simulink model "AFASClosedloopSim"  (R2023a)
settings: Solver=FixedStepAuto  StartTime=0.0  StopTime=600  FixedStep=1/240  RelTol=1e-5
PreLoadFcn:
  | [aircraft, state] = astDehavillandBeaver();
  | thrustX = getCoefficient(aircraft,"CX","Propeller",Component="Propeller");
InitFcn:
  | AFASClosedloopSimInitialization
model workspace (MATLAB code in the model file + MAT data in the model file):
  AirReferencedVelocity = 1
  AircraftPerformance : object (value not decoded)
  CurrentWaypoint = 1
  FCCLatDirMode = 1
  FCCVerticalMode = 1
  FlightPlan = 1
  LookaheadDis = 15
  NextWaypoint = 1
  NumofWaypoint = 1
  OwnshipAircraftID = 1
  PreWaypoint = 1
  PreviousWaypoint : Simulink.Parameter (value not decoded)
  TrajectoryChange = 1
  WaypointType = 1
  inputs0 : object (value not decoded)
  states : object (value not decoded)
  states0 : object (value not decoded)
  other statements: initialize6DOFSkyHogg;
values from neighbouring files (symbols this model uses):
  alt_ft = 1000    [AFASClosedloopSimInitialization.m]
  alt_hold_av = 1.5    [AFASClosedloopSimInitialization.m]
  alt_hold_hold = 0.1    [AFASClosedloopSimInitialization.m]
  alt_hold_vs = 0.58    [AFASClosedloopSimInitialization.m]
  alt_m = 304.8    [AFASClosedloopSimInitialization.m]
  AT_lead_T1 = 1    [AFASClosedloopSimInitialization.m]
  AT_lead_T2 = 1    [AFASClosedloopSimInitialization.m]
  AT_spd_hold_cmpst = 0.5    [AFASClosedloopSimInitialization.m]
  AT_spd_hold_ptch_tau_gain = 0.15    [AFASClosedloopSimInitialization.m]
  AT_spd_hold_rate_damping_gain = 10    [AFASClosedloopSimInitialization.m]
  AT_spd_hold_tas_lp_tau = 5.0    (= 5)    [AFASClosedloopSimInitialization.m]
  AT_spd_hold_tas_val_lp_tau = 0.5    [AFASClosedloopSimInitialization.m]
  AT_struct_den = 1    [AFASClosedloopSimInitialization.m]
  AT_struct_num = 1    [AFASClosedloopSimInitialization.m]
  AT_svo_composite = 1    [AFASClosedloopSimInitialization.m]
  av_hp_fltr_tau = 10    [AFASClosedloopSimInitialization.m]
  av_lp_fltr_tau = 0.5    [AFASClosedloopSimInitialization.m]
  cas_mps = 72.0222    [AFASClosedloopSimInitialization.m]
  Cl0 = 5.910000000000000e-04    (= 0.000591)    [AFASClosedloopSimInitialization.m]
  Cl_beta = -0.0618    [AFASClosedloopSimInitialization.m]
  Cl_da = -0.0992    [AFASClosedloopSimInitialization.m]
  Cl_da_alpha = -0.0827    [AFASClosedloopSimInitialization.m]
  Cl_dr = 0.0069    [AFASClosedloopSimInitialization.m]
  Cl_p = -0.5045    [AFASClosedloopSimInitialization.m]
  Cl_r = 0.1695    [AFASClosedloopSimInitialization.m]
  Cm0 = 0.0945    [AFASClosedloopSimInitialization.m]
  Cm_alpha = -0.6028    [AFASClosedloopSimInitialization.m]
  Cm_alpha2 = -2.1400    (= -2.14)    [AFASClosedloopSimInitialization.m]
  Cm_beta2 = 0.6921    [AFASClosedloopSimInitialization.m]
  Cm_de = -1.9210    (= -1.921)    [AFASClosedloopSimInitialization.m]
  Cm_df = 0.4072    [AFASClosedloopSimInitialization.m]
  Cm_q = -15.5600    (= -15.56)    [AFASClosedloopSimInitialization.m]
  Cm_r = -0.3118    [AFASClosedloopSimInitialization.m]
  Cn0 = -0.0031    [AFASClosedloopSimInitialization.m]
  Cn_beta = 0.0067    [AFASClosedloopSimInitialization.m]
  Cn_beta3 = 0.1373    [AFASClosedloopSimInitialization.m]
  Cn_da = -0.0039    [AFASClosedloopSimInitialization.m]
  Cn_dr = -0.0827    [AFASClosedloopSimInitialization.m]
  Cn_p = -0.1585    [AFASClosedloopSimInitialization.m]
  Cn_q = 0.1595    [AFASClosedloopSimInitialization.m]
  Cn_r = -0.1112    [AFASClosedloopSimInitialization.m]
  Cx0 = -0.0355    [AFASClosedloopSimInitialization.m]
  Cx_alpha = 0.0029    [AFASClosedloopSimInitialization.m]
  Cx_alpha2 = 5.4590    (= 5.459)    [AFASClosedloopSimInitialization.m]
  Cx_alpha3 = -5.1620    (= -5.162)    [AFASClosedloopSimInitialization.m]
  Cx_df = -0.0945    [AFASClosedloopSimInitialization.m]
  Cx_df_alpha = 1.1060    (= 1.106)    [AFASClosedloopSimInitialization.m]
  Cx_dr = 0.0341    [AFASClosedloopSimInitialization.m]
  Cx_q = -0.6748    [AFASClosedloopSimInitialization.m]
  Cy0 = -0.0022    [AFASClosedloopSimInitialization.m]
  Cy_beta = -0.7678    [AFASClosedloopSimInitialization.m]
  Cy_da = -0.0296    [AFASClosedloopSimInitialization.m]
  Cy_dr = 0.1158    [AFASClosedloopSimInitialization.m]
  Cy_dr_alpha = 0.5238    [AFASClosedloopSimInitialization.m]
  Cy_p = -0.1240    (= -0.124)    [AFASClosedloopSimInitialization.m]
  Cy_r = 0.3666    [AFASClosedloopSimInitialization.m]
  Cz0 = -0.0550    (= -0.055)    [AFASClosedloopSimInitialization.m]
  Cz_alpha = -5.5780    (= -5.578)    [AFASClosedloopSimInitialization.m]
  Cz_alpha3 = 3.4420    (= 3.442)    [AFASClosedloopSimInitialization.m]
  Cz_de = -0.3980    (= -0.398)    [AFASClosedloopSimInitialization.m]
  Cz_de_beta = -15.9300    (= -15.93)    [AFASClosedloopSimInitialization.m]
  Cz_df = -1.3770    (= -1.377)    [AFASClosedloopSimInitialization.m]
  Cz_df_alpha = -1.2610    (= -1.261)    [AFASClosedloopSimInitialization.m]
  Cz_q = -2.9880    (= -2.988)    [AFASClosedloopSimInitialization.m]
  hdg_select_hdg_rate_capt = 0.2    [AFASClosedloopSimInitialization.m]
  hdg_select_hdg_rate_damping = 1    [AFASClosedloopSimInitialization.m]
  hdg_select_hdg_rate_track = 0.05    [AFASClosedloopSimInitialization.m]
  lat_accel_aug_lp_tau = 10    [AFASClosedloopSimInitialization.m]
  ltrl_acc_gain = -0.04    [AFASClosedloopSimInitialization.m]
  ltrl_acc_lp_tau = 0.5    [AFASClosedloopSimInitialization.m]
  mach = 0.213    [AFASClosedloopSimInitialization.m]
  OwnshipAircraftConfig = 0    [AFASClosedloopSimInitialization.m]
  pitch_att_gain = 0.7    [AFASClosedloopSimInitialization.m]
  pitch_lead_T1 = 1    [AFASClosedloopSimInitialization.m]
  pitch_lead_T2 = 1    [AFASClosedloopSimInitialization.m]
  pitch_rate_gain = -1400    [AFASClosedloopSimInitialization.m]
  pitch_rate_gain_GAIN1 = -56    [AFASClosedloopSimInitialization.m]
  pitch_rate_gain_GAIN2 = -52.25    [AFASClosedloopSimInitialization.m]
  pitch_rate_gain_IAS1 = 100    [AFASClosedloopSimInitialization.m]
  pitch_rate_gain_IAS2 = 380    [AFASClosedloopSimInitialization.m]
  pitch_rate_gain_schd = [4.24        2.80        2.24        1.68        1.44        1.22        0.97        0.85        0.77        0.72        0.66    ] * 1000    [AFASClosedloopSimInitialization.m]
  pitch_rate_gain_spd = [85          100.0       120.00      140.00      160.00      180.00      200.00      220.00      240.00      260.00      275.00  ] * 0.5144444    [AFASClosedloopSimInitialization.m]
  pitch_schedule_type = 3    [AFASClosedloopSimInitialization.m]
  pitch_struct_den = 1    [AFASClosedloopSimInitialization.m]
  pitch_struct_num = 1    [AFASClosedloopSimInitialization.m]
  pitch_svo_composite = 1    [AFASClosedloopSimInitialization.m]
  pitch_svo_integral = 0.6    [AFASClosedloopSimInitialization.m]
  roll_att_gain = 0.45    [AFASClosedloopSimInitialization.m]
  roll_lead_T1 = 1    [AFASClosedloopSimInitialization.m]
  roll_lead_T2 = 1    [AFASClosedloopSimInitialization.m]
  roll_limit = 30*d2r    (= 0.5235987)    [AFASClosedloopSimInitialization.m]
  roll_rate_gain = 561.5    [AFASClosedloopSimInitialization.m]
  roll_rate_gain_GAIN1 = 57.25    [AFASClosedloopSimInitialization.m]
  roll_rate_gain_GAIN2 = 41.25    [AFASClosedloopSimInitialization.m]
  roll_rate_gain_IAS1 = 100    [AFASClosedloopSimInitialization.m]
  roll_rate_gain_IAS2 = 380    [AFASClosedloopSimInitialization.m]
  roll_rate_gain_schd = [1.30        0.86        0.71        0.63        0.57        0.50        0.46        0.46    ] * 1000    [AFASClosedloopSimInitialization.m]
  roll_rate_gain_spd = [85.00       100.00      120.00      140.00      160.00      200.00      220.00      275.00  ] * 0.5144444    [AFASClosedloopSimInitialization.m]
  roll_schedule_type = 3    [AFASClosedloopSimInitialization.m]
  roll_struct_den = 1    [AFASClosedloopSimInitialization.m]
  roll_struct_num = 1    [AFASClosedloopSimInitialization.m]
  roll_svo_composite = 0.00001    (= 1e-05)    [AFASClosedloopSimInitialization.m]
  roll_svo_integral = 0.6    [AFASClosedloopSimInitialization.m]
  tas_mps = 73.051    [AFASClosedloopSimInitialization.m]
  TGR = 0.25    [AFASClosedloopSimInitialization.m]
  wingrock_enable_alt = 20000    [AFASClosedloopSimInitialization.m]
  wingrock_enable_mach = 0.6    [AFASClosedloopSimInitialization.m]
  wingrock_lookup_data = [2 2  1 1]    [AFASClosedloopSimInitialization.m]
  wingrock_lookup_row = [0 2 5 10]*pi/180    [AFASClosedloopSimInitialization.m]
  wingrock_schedule_type = 3    [AFASClosedloopSimInitialization.m]
  yaw_rate_gain = 15521    [AFASClosedloopSimInitialization.m]
  yaw_rate_gain_GAIN1 = 37.8352    [AFASClosedloopSimInitialization.m]
  yaw_rate_gain_GAIN2 = 24.2654    [AFASClosedloopSimInitialization.m]
  yaw_rate_gain_IAS1 = 100    [AFASClosedloopSimInitialization.m]
  yaw_rate_gain_IAS2 = 340    [AFASClosedloopSimInitialization.m]
  yaw_rate_gain_piecewise_schd = [7.68	5.98		3.22	2.59		1.78 ... (first row only)    [AFASClosedloopSimInitialization.m]
  yaw_rate_gain_schd = [15521    11532   11532   10115   8951.7  7831.7  6829.2  5739.3  4506.7  3317.9  3391.5  2103.9  1404.5  994.3226]    [AFASClosedloopSimInitialization.m]
  yaw_rate_gain_spd = [90       97      106     111     118     127     136     149     165     187     192     228     264     295     ] * 0.5144444    [AFASClosedloopSimInitialization.m]
  yaw_rate_hp_tau = 1.8    [AFASClosedloopSimInitialization.m]
  yd_lead_T1 = yd_a * yd_lead_T2    [AFASClosedloopSimInitialization.m]
  ... (+7 more)
undefined symbols (not defined in the file or in its folder): aircraft, DiscIntNeverNeededParam, Earth, F, Light, MIL, sigbuilder_block, state, WGS84
libraries: aerolibasang x4, aerolibactuator x4, aerolibguid x2, simulink x2, dspnetwork x2, etargetslib x2, shared6dof x1, aerolibadyn x1, aerolibatmos2 x1, aerolibwind2 x1, aerolibtransform2 x1, sharedtransform x1
(part 4 of 4)

== system AFASClosedloopSim/FMGC (Flight Mgt and Guidance & Control)/AFCC: Albatross.ai Flight Control Computer/FCC: Outerloop & Innerloop Control Laws/HDG Mode/Outerloop Control Law ==
  psiCmd_rad : Inport
  psiF_rad : Inport  Port=2
  psiDotF_rps : Inport  Port=3
  "phiF_rad " : Inport  Port=4
  "phiDotF_rps " : Inport  Port=5
  rF_rps : Inport  Port=6
  "AyF_mpss " : Inport  Port=7
  Constant : Constant  Value=tas_mps
      settings: AttributesFormatString=TAS_mps
  HDG Flight Director : Subsystem
  Manual Switch4 : ManualSwitch  CurrentSetting=0
  Outerloop AP Delay{,1..3} (4 alike) : TransportDelay  DelayTime=0.004
  Outerloop FD Delay : TransportDelay  DelayTime=0.0905
  PFD/MFD Delay1 : TransportDelay  DelayTime=0.0175
  PFD/MFD Delay2 : TransportDelay  DelayTime=0.0175
  PFD/MFD Delay3 : TransportDelay  DelayTime=0.0175
  Roll Command Ay Augmentation : Subsystem
  Scope1 : Scope
  Scope2 : Scope
  Subsystem1 : Subsystem  mask(Zero-Order Hold){Tau=0.025}
      mask prompts: Tau "Tau (s)"
      mask help: Zero-Order Hold
      settings: AttributesFormatString=ZOH\n
      mask Display: disp([num2str(1/Tau),'Hz'])
  Subsystem2 : Subsystem  mask(Zero-Order Hold){Tau=0.025}
      mask prompts: Tau "Tau (s)"
      mask help: Zero-Order Hold
      settings: AttributesFormatString=ZOH\n
      mask Display: disp([num2str(1/Tau),'Hz'])
  Subsystem3 : Subsystem  mask(Zero-Order Hold){Tau=0.025}
      mask prompts: Tau "Tau (s)"
      mask help: Zero-Order Hold
      settings: AttributesFormatString=ZOH\n
      mask Display: disp([num2str(1/Tau),'Hz'])
  Subsystem4 : Subsystem  mask(Zero-Order Hold){Tau=0.025}
      mask prompts: Tau "Tau (s)"
      mask help: Zero-Order Hold
      settings: AttributesFormatString=ZOH\n
      mask Display: disp([num2str(1/Tau),'Hz'])
  Subsystem5 : Subsystem  mask(Zero-Order Hold){Tau=0.1000}
      mask prompts: Tau "Tau (s)"
      mask help: Zero-Order Hold
      settings: AttributesFormatString=ZOH\n
      mask Display: disp([num2str(1/Tau),'Hz'])
  Sum : Sum  Inputs=|++  SaturateOnIntegerOverflow=on
  hdg_select : Subsystem
  phiCmd_rad : Outport  InitialOutput=0
  phiC_rad : Outport  Port=2
  rC_rps : Outport  Port=3
  AyC_mpss : Outport  Port=4
  phiDotC_rps : Outport  Port=5
  wires:
  HDG Flight Director/1(phiCmd_rad) -> Manual Switch4/2
  "phiF_rad "/1 -> Outerloop AP Delay1/1
  "phiDotF_rps "/1 -> Outerloop AP Delay3/1
  rF_rps/1 -> Outerloop AP Delay2/1
  "AyF_mpss "/1 -> Outerloop AP Delay/1, PFD/MFD Delay3/1
  Subsystem5/1(Out) -> Scope2/1, phiCmd_rad/1
  Outerloop AP Delay2/1 -> Subsystem3/1(In)
  Subsystem4/1(Out) -> AyC_mpss/1
  Subsystem1/1(Out) -> phiC_rad/1
  Subsystem2/1(Out) -> phiDotC_rps/1
  Subsystem3/1(Out) -> rC_rps/1
  Outerloop AP Delay/1 -> Subsystem4/1(In)
  Outerloop AP Delay3/1 -> Subsystem2/1(In)
  Outerloop AP Delay1/1 -> Subsystem1/1(In)
  PFD/MFD Delay2/1 -> HDG Flight Director/2(psi_rad), hdg_select/2(hdg)
  PFD/MFD Delay3/1 -> Roll Command Ay Augmentation/1(AyAHF_m)
  Outerloop FD Delay/1 -> Subsystem5/1(In)
  psiDotF_rps/1 -> PFD/MFD Delay1/1
  PFD/MFD Delay1/1 -> HDG Flight Director/3(psiDot_rps), hdg_select/4(hdg_rate)
  Sum/1 -> Outerloop FD Delay/1
  Roll Command Ay Augmentation/1(augCmd_rad) -> Sum/2
  psiCmd_rad/1 -> Scope1/1, HDG Flight Director/1(psiCmd_rad), hdg_select/1(slctd_hdg)
  Constant/1 -> hdg_select/3(tas)
  hdg_select/1(roll_cmd) -> Manual Switch4/1
  Manual Switch4/1 -> Sum/1
  psiF_rad/1 -> PFD/MFD Delay2/1

== system AFASClosedloopSim/FMGC (Flight Mgt and Guidance & Control)/AFCC: Albatross.ai Flight Control Computer/FCC: Outerloop & Innerloop Control Laws/ALT Mode/Innerloop Control Law/Autopilot IAS-scheduled Gain ==
  ias : Inport
  Gain Sign : Constant  Value=-1
  Look-Up Table : Lookup  InputValues="[ias_1  ias_2]"  Table="[abs_gain_1  abs_gain_2]"  LookUpMeth=Interpolation-Use End Values
  Product : Product  InputSameDT=on  SaturateOnIntegerOverflow=on  OutDataTypeStr=Inherit: Same as first input
  dB->linear : Fcn  Expr=2^(u(1)/8)
  scheduled_gain : Outport
  wires:
  Gain Sign/1 -> Product/2
  Product/1 -> scheduled_gain/1
  ias/1 -> Look-Up Table/1
  dB->linear/1 -> Product/1
  Look-Up Table/1 -> dB->linear/1

== system AFASClosedloopSim/FMGC (Flight Mgt and Guidance & Control)/AFCC: Albatross.ai Flight Control Computer/FCC: Outerloop & Innerloop Control Laws/ALT Mode/Outerloop Control Law/Alt Upset_m ==
  Demux : Demux  Tag=STV Demux  Outputs=1
      settings: DisplayOption=none
  FromWs : FromWorkspace  Tag=STV FromWs  VariableName=tuvar
      SigBuilderData=|
      | common.afterFinalStr = 'Extrapolate'
      | common.sampleTime = 0
      | dataSet.timeRange = [0 50]
      | dataSet.name = 'Group 1'
      | sbobj.Groups.Name = 'Group 1'
      | sbobj.Groups.Signals.Name = 'Signal 2'
      | sbobj.Groups.Signals.XData = [0 5 5 6 6 50]
      | sbobj.Groups.Signals.YData = [0 0 5 5 0 0]
      | sbobj.Groups.TimeRange = [0 50]
  Signal 2 : Outport  Tag=STV Outport
  wires:
  Demux/1 -> Signal 2/1
  FromWs/1 -> Demux/1

== system AFASClosedloopSim/FMGC (Flight Mgt and Guidance & Control)/AFCC: Albatross.ai Flight Control Computer/FCC: Outerloop & Innerloop Control Laws/ALT Mode/Outerloop Control Law/Complementary Filter ==
  hd_mps : Inport
  hdd_mpss : Inport  Port=2
  " Av_HP" : TransferFcn  Numerator=[1 0]  Denominator=[av_hp_fltr_tau 1]
  " HP Filter  " : TransferFcn  Numerator=[1.2596 2.0202]  Denominator=[1.2596 2.0202 1]
  HP Filter : TransferFcn  Numerator=[1.2596 2.0202]  Denominator=[1.2596 2.0202 1]
  Sum1 : Sum  Inputs=++|  SaturateOnIntegerOverflow=on
  Sum2 : Sum  Inputs=|++  SaturateOnIntegerOverflow=on
  Sum3 : Sum  Inputs=++|  SaturateOnIntegerOverflow=on
  av_hp_fltr_tau : Gain  Gain=av_hp_fltr_tau  SaturateOnIntegerOverflow=on  OutDataTypeStr=Inherit: Same as input  ParamDataTypeStr=Inherit: Same as input
  hdF_mps : Outport
  hddF_mpss : Outport  Port=2
  wires:
  hdd_mpss/1 -> HP Filter/1, av_hp_fltr_tau/1
  hd_mps/1 -> Sum1/1, Sum3/1
  Sum2/1 -> Sum3/2
  HP Filter/1 -> Sum2/1
  av_hp_fltr_tau/1 -> Sum2/2
  Sum1/1 -> hdF_mps/1
  " HP Filter  "/1 -> Sum1/2
  " Av_HP"/1 -> " HP Filter  "/1, hddF_mpss/1
  Sum3/1 -> " Av_HP"/1

== system AFASClosedloopSim/FMGC (Flight Mgt and Guidance & Control)/AFCC: Albatross.ai Flight Control Computer/FCC: Outerloop & Innerloop Control Laws/ALT Mode/Outerloop Control Law/Subsystem ==
  In : Inport
  ZOH : TransferFcn  Numerator=[-Tau/6 1]  Denominator=[Tau/3 1]
  Out : Outport
  wires:
  ZOH/1 -> Out/1
  In/1 -> ZOH/1

== system AFASClosedloopSim/FMGC (Flight Mgt and Guidance & Control)/AFCC: Albatross.ai Flight Control Computer/FCC: Outerloop & Innerloop Control Laws/ALT Mode/Outerloop Control Law/Subsystem1 ==
  In : Inport
  ZOH : TransferFcn  Numerator=[-Tau/6 1]  Denominator=[Tau/3 1]
  Out : Outport
  wires:
  In/1 -> ZOH/1
  ZOH/1 -> Out/1

== system AFASClosedloopSim/FMGC (Flight Mgt and Guidance & Control)/AFCC: Albatross.ai Flight Control Computer/FCC: Outerloop & Innerloop Control Laws/ALT Mode/Outerloop Control Law/VS Upset_fpm ==
  Demux : Demux  Tag=STV Demux  Outputs=1
      settings: DisplayOption=none
  FromWs : FromWorkspace  Tag=STV FromWs  VariableName=tuvar
      SigBuilderData=|
      | common.afterFinalStr = 'Extrapolate'
      | common.sampleTime = 0
      | dataSet.timeRange = [0 50]
      | dataSet.name = 'Group 1'
      | sbobj.Groups.Name = 'Group 1'
      | sbobj.Groups.Signals.Name = 'Signal 2'
      | sbobj.Groups.Signals.XData = [0 5 5 6 6 50]
      | sbobj.Groups.Signals.YData = [0 0 200 200 0 0]
      | sbobj.Groups.TimeRange = [0 50]
  Signal 2 : Outport  Tag=STV Outport
  wires:
  FromWs/1 -> Demux/1
  Demux/1 -> Signal 2/1

== system AFASClosedloopSim/FMGC (Flight Mgt and Guidance & Control)/AFCC: Albatross.ai Flight Control Computer/FCC: Outerloop & Innerloop Control Laws/Autothrottle/AT SPD Hold//Select/Subsystem ==
  In : Inport
  ZOH : TransferFcn  Numerator=[-Tau/6 1]  Denominator=[Tau/3 1]
  Out : Outport
  wires:
  ZOH/1 -> Out/1
  In/1 -> ZOH/1

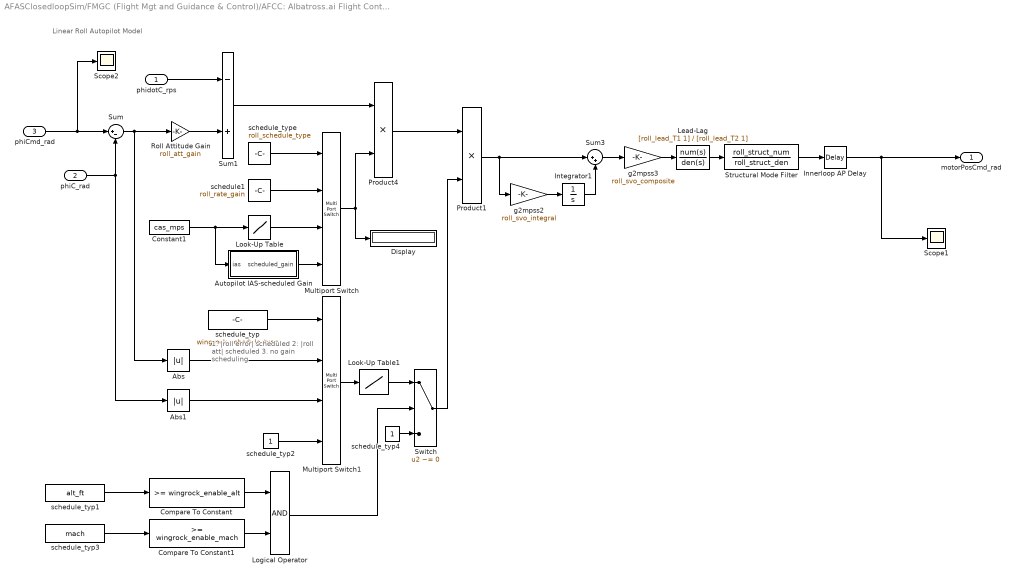
== system AFASClosedloopSim/FMGC (Flight Mgt and Guidance & Control)/AFCC: Albatross.ai Flight Control Computer/FCC: Outerloop & Innerloop Control Laws/HDG Mode/Innerloop Control Law/Roll AP ==
  note: Linear Roll Autopilot Model
  note: 1: |roll error| scheduled
      | 2: |roll att| scheduled
      | 3. no gain scheduling
  phidotC_rps : Inport
  phiC_rad : Inport  Port=2
  phiCmd_rad : Inport  Port=3
  Abs : Abs  SaturateOnIntegerOverflow=off
  Abs1 : Abs  SaturateOnIntegerOverflow=off
  Autopilot IAS-scheduled Gain : Subsystem  mask(Autopilot IAS-scheduled Gain){IAS1=roll_rate_gain_IAS1, IAS2=roll_rate_gain_IAS2, GAIN1=roll_rate_gain_GAIN1, GAIN2=roll_rate_gain_GAIN2}
      mask prompts: IAS1 "IAS1 (lower IAS limit, knots)"; IAS2 "IAS2 (upper IAS limit, knots)"; GAIN1 "GAIN1 (the gain for IAS1, dB)"; GAIN2 "GAIN2 (the gain for IAS2, dB)"
      mask help:
      | Autopilot gain scheduling based on the indicated airspeed.
      |
      | Parameters:
      | IAS1 (lower IAS limit, knots)  -- lower IAS limit (unit: knot)
      | IAS2 (upper IAS limit, knots) -- upper IAS limit (unit: knot)
      | GAIN1 (the gain for IAS1, dB) -- the gain for the lower IAS limit (unit: dB)
      | GAIN2 (the gain for IAS2, dB) -- the gain for the upper IAS limit (unit: dB)
      |
      | Inputs:
      | ias -- indicated airspeed (unit: meter/second)
      |
      | Outputs:
      | scheduled_gain -- indicated airspeed scheduled gain
      mask init:
      | ias_1 = IAS1 * 0.5144444;
      | ias_2 = IAS2 * 0.5144444;
      | abs_gain_1 = abs( GAIN1 ) * 8 / 6;
      | abs_gain_2 = abs( GAIN2 ) * 8 / 6;
      | gain_sign = sign( GAIN1 );
      mask Help:
      | Autopilot gain scheduling based on the indicated airspeed.
      | 
      | Parameters:
      | IAS1 (lower IAS limit, knots)  -- lower IAS limit (unit: knot)
      | IAS2 (upper IAS limit, knots) -- upper IAS limit (unit: knot)
      | GAIN1 (the gain for IAS1, dB) -- the gain for the lower IAS limit (unit: dB)
      | GAIN2 (the gain for IAS2, dB) -- the gain for the upper IAS limit (unit: dB)
      | 
      | Inputs:
      | ias -- indicated airspeed (unit: meter/second)
      | 
      | Outputs:
      | scheduled_gain -- indicated airspeed scheduled gain
  Compare To Constant : simulink/Logic and Bit Operations/Compare To Constant  relop=>=  const=wingrock_enable_alt  OutDataTypeStr=boolean
  Compare To Constant1 : simulink/Logic and Bit Operations/Compare To Constant  relop=>=  const=wingrock_enable_mach  OutDataTypeStr=boolean
  Constant1 : Constant  Value=cas_mps
      settings: AttributesFormatString=CAS_mps
  Display : Display
  Innerloop AP Delay : TransportDelay  DelayTime=0.003
  Integrator1 : Integrator
  Lead-Lag : TransferFcn  Numerator=[roll_lead_T1 1]  Denominator=[roll_lead_T2 1]
  Logical Operator : Logic  AllPortsSameDT=off  OutDataTypeStr=boolean
  Look-Up Table : Lookup  InputValues=roll_rate_gain_spd  Table=roll_rate_gain_schd  LookUpMeth=Interpolation-Use End Values
  Look-Up Table1 : Lookup  InputValues=wingrock_lookup_row  Table=wingrock_lookup_data  LookUpMeth=Interpolation-Use End Values
  Multiport Switch : MultiPortSwitch  InputSameDT=off
  Multiport Switch1 : MultiPortSwitch  InputSameDT=off
  Product1 : Product  Inputs=**  InputSameDT=on  SaturateOnIntegerOverflow=on  OutDataTypeStr=Inherit: Same as first input
  Product4 : Product  Inputs=**  InputSameDT=on  SaturateOnIntegerOverflow=on  OutDataTypeStr=Inherit: Same as first input
  Roll Attitude Gain : Gain  Gain=roll_att_gain  SaturateOnIntegerOverflow=on  OutDataTypeStr=Inherit: Same as input  ParamDataTypeStr=Inherit: Same as input
      settings: AttributesFormatString=%<Gain>
  Scope1 : Scope
  Scope2 : Scope
  Structural Mode Filter : TransferFcn  Numerator=roll_struct_num  Denominator=roll_struct_den
  Sum : Sum  Inputs=|+-  SaturateOnIntegerOverflow=on
  Sum1 : Sum  Inputs=-+  SaturateOnIntegerOverflow=on
  Sum3 : Sum  Inputs=|++  SaturateOnIntegerOverflow=on
  Switch : Switch  Criteria=u2 ~= 0  SaturateOnIntegerOverflow=off  InputSameDT=off
  g2mpss2 : Gain  Gain=roll_svo_integral  SaturateOnIntegerOverflow=on  OutDataTypeStr=Inherit: Same as input  ParamDataTypeStr=Inherit: Same as input
  g2mpss3 : Gain  Gain=roll_svo_composite  SaturateOnIntegerOverflow=on  OutDataTypeStr=Inherit: Same as input  ParamDataTypeStr=Inherit: Same as input
  schedule1 : Constant  Value=roll_rate_gain
      settings: AttributesFormatString=roll_rate_gain
  schedule_typ : Constant  Value=wingrock_schedule_type
  schedule_typ1 : Constant  Value=alt_ft
  schedule_typ2 : Constant
  schedule_typ3 : Constant  Value=mach
  schedule_typ4 : Constant
  schedule_type : Constant  Value=roll_schedule_type
  motorPosCmd_rad : Outport
  wires:
  Sum1/1 -> Product4/1
  Roll Attitude Gain/1 -> Sum1/2
  Innerloop AP Delay/1 -> Scope1/1, motorPosCmd_rad/1
  Structural Mode Filter/1 -> Innerloop AP Delay/1
  Multiport Switch/1 -> Product4/2, Display/1
  Constant1/1 -> Autopilot IAS-scheduled Gain/1(ias), Look-Up Table/1
  schedule1/1 -> Multiport Switch/2
  Look-Up Table/1 -> Multiport Switch/3
  schedule_type/1 -> Multiport Switch/1
  Autopilot IAS-scheduled Gain/1(scheduled_gain) -> Multiport Switch/4
  Sum/1 -> Roll Attitude Gain/1, Abs/1
  Integrator1/1 -> Sum3/2
  g2mpss2/1 -> Integrator1/1
  Sum3/1 -> g2mpss3/1
  phiCmd_rad/1 -> Scope2/1, Sum/1
  phiC_rad/1 -> Sum/2, Abs1/1
  schedule_typ/1 -> Multiport Switch1/1
  schedule_typ2/1 -> Multiport Switch1/4
  schedule_typ1/1 -> Compare To Constant/1
  schedule_typ3/1 -> Compare To Constant1/1
  Compare To Constant/1 -> Logical Operator/1
  Compare To Constant1/1 -> Logical Operator/2
  Multiport Switch1/1 -> Look-Up Table1/1
  Logical Operator/1 -> Switch/2
  Look-Up Table1/1 -> Switch/1
  schedule_typ4/1 -> Switch/3
  Switch/1 -> Product1/2
  Product4/1 -> Product1/1
  Product1/1 -> Sum3/1, g2mpss2/1
  g2mpss3/1 -> Lead-Lag/1
  Lead-Lag/1 -> Structural Mode Filter/1
  phidotC_rps/1 -> Sum1/1
  Abs/1 -> Multiport Switch1/2
  Abs1/1 -> Multiport Switch1/3

== system AFASClosedloopSim/FMGC (Flight Mgt and Guidance & Control)/AFCC: Albatross.ai Flight Control Computer/FCC: Outerloop & Innerloop Control Laws/HDG Mode/Innerloop Control Law/YD Control Law ==
  phiC_rad : Inport
  rC_rps : Inport  Port=2
  AyC_mpss : Inport  Port=3
  Attitude Gain1 : Gain  Gain=ltrl_acc_gain  SaturateOnIntegerOverflow=on  OutDataTypeStr=Inherit: Same as input  ParamDataTypeStr=Inherit: Same as input
      settings: AttributesFormatString=%<Gain>
  Autopilot IAS-scheduled Gain : Subsystem  mask(Autopilot IAS-scheduled Gain){IAS1=yaw_rate_gain_IAS1, IAS2=yaw_rate_gain_IAS2, GAIN1=yaw_rate_gain_GAIN1, GAIN2=yaw_rate_gain_GAIN2}
      mask prompts: IAS1 "IAS1 (lower IAS limit, knots)"; IAS2 "IAS2 (upper IAS limit, knots)"; GAIN1 "GAIN1 (the gain for IAS1, dB)"; GAIN2 "GAIN2 (the gain for IAS2, dB)"
      mask help:
      | Autopilot gain scheduling based on the indicated airspeed.
      |
      | Parameters:
      | IAS1 (lower IAS limit, knots)  -- lower IAS limit (unit: knot)
      | IAS2 (upper IAS limit, knots) -- upper IAS limit (unit: knot)
      | GAIN1 (the gain for IAS1, dB) -- the gain for the lower IAS limit (unit: dB)
      | GAIN2 (the gain for IAS2, dB) -- the gain for the upper IAS limit (unit: dB)
      |
      | Inputs:
      | ias -- indicated airspeed (unit: meter/second)
      |
      | Outputs:
      | scheduled_gain -- indicated airspeed scheduled gain
      mask init:
      | ias_1 = IAS1 * 0.5144444;
      | ias_2 = IAS2 * 0.5144444;
      | abs_gain_1 = abs( GAIN1 ) * 8 / 6;
      | abs_gain_2 = abs( GAIN2 ) * 8 / 6;
      | gain_sign = sign( GAIN1 );
      mask Help:
      | Autopilot gain scheduling based on the indicated airspeed.
      | 
      | Parameters:
      | IAS1 (lower IAS limit, knots)  -- lower IAS limit (unit: knot)
      | IAS2 (upper IAS limit, knots) -- upper IAS limit (unit: knot)
      | GAIN1 (the gain for IAS1, dB) -- the gain for the lower IAS limit (unit: dB)
      | GAIN2 (the gain for IAS2, dB) -- the gain for the upper IAS limit (unit: dB)
      | 
      | Inputs:
      | ias -- indicated airspeed (unit: meter/second)
      | 
      | Outputs:
      | scheduled_gain -- indicated airspeed scheduled gain
  CAS_mps : Constant  Value=cas_mps
  CAS_mps1 : Constant  Value=cas_mps
  Display : Display
  Innerloop AP Delay : TransportDelay  DelayTime=0.003
  Integrator1 : Integrator
  Lead-Lag : TransferFcn  Numerator=[yd_lead_T1 1]  Denominator=[yd_lead_T2 1]
  Look-Up Table : Lookup  InputValues=yaw_rate_gain_spd  Table=yaw_rate_gain_schd  LookUpMeth=Interpolation-Use End Values
  Lookup Table (2-D) : Lookup2D  RowIndex=yaw_rate_gain_piecewise_alt  ColumnIndex=yaw_rate_gain_piecewise_spd  Table=yaw_rate_gain_piecewise_schd  LookUpMeth=Interpolation-Use End Values  SaturateOnIntegerOverflow=off  InputSameDT=off
  Multiport Switch : MultiPortSwitch  Inputs=4  InputSameDT=off
  Product : Product  Inputs=*/  InputSameDT=on  SaturateOnIntegerOverflow=on  OutDataTypeStr=Inherit: Same as first input
  Product3 : Product  Inputs=**  InputSameDT=on  SaturateOnIntegerOverflow=on  OutDataTypeStr=Inherit: Same as first input
  Structural Mode Filter : TransferFcn  Numerator=yd_struct_num  Denominator=yd_struct_den
  Sum1 : Sum  Inputs=--  SaturateOnIntegerOverflow=on
  Sum2 : Sum  Inputs=+-  SaturateOnIntegerOverflow=on
  Sum3 : Sum  Inputs=|++  SaturateOnIntegerOverflow=on
  Transfer Fcn1 : TransferFcn  Numerator=1  Denominator=[ltrl_acc_lp_tau 1]
      settings: AttributesFormatString=1/(tau*s+1)
  Transfer Fcn2 : TransferFcn  Numerator="[yaw_rate_hp_tau   0]"  Denominator="[yaw_rate_hp_tau   1]"
      settings: AttributesFormatString=(tau*s) / (tau*s+1)
  alt_m : Constant  Value=alt_m
  g2mpss : Gain  Gain=9.80665  SaturateOnIntegerOverflow=on  OutDataTypeStr=Inherit: Same as input  ParamDataTypeStr=Inherit: Same as input
      settings: AttributesFormatString=g2mpss
  g2mpss1 : Gain  Gain=yd_svo_integral  SaturateOnIntegerOverflow=on  OutDataTypeStr=Inherit: Same as input  ParamDataTypeStr=Inherit: Same as input
  g2mpss2 : Gain  Gain=yd_svo_composite  SaturateOnIntegerOverflow=on  OutDataTypeStr=Inherit: Same as input  ParamDataTypeStr=Inherit: Same as input
  schedule1 : Constant  Value=yaw_rate_gain
      settings: AttributesFormatString=yaw_rate_gain
  schedule_type : Constant  Value=yd_schedule_type
  motorPosCmd_rad : Outport  InitialOutput=0
  wires:
  phiC_rad/1 -> Product/1
  Product/1 -> g2mpss/1
  AyC_mpss/1 -> Attitude Gain1/1
  Innerloop AP Delay/1 -> motorPosCmd_rad/1
  Sum2/1 -> Transfer Fcn2/1
  schedule1/1 -> Multiport Switch/2
  Sum1/1 -> Product3/1
  Look-Up Table/1 -> Multiport Switch/3
  Multiport Switch/1 -> Display/1, Product3/2
  Autopilot IAS-scheduled Gain/1(scheduled_gain) -> Multiport Switch/4
  schedule_type/1 -> Multiport Switch/1
  Structural Mode Filter/1 -> Innerloop AP Delay/1
  Product3/1 -> g2mpss1/1, Sum3/1
  CAS_mps1/1 -> Lookup Table (2-D)/2, Autopilot IAS-scheduled Gain/1(ias), Look-Up Table/1
  Integrator1/1 -> Sum3/2
  g2mpss1/1 -> Integrator1/1
  Sum3/1 -> g2mpss2/1
  g2mpss2/1 -> Lead-Lag/1
  CAS_mps/1 -> Product/2
  Lookup Table (2-D)/1 -> Multiport Switch/5
  alt_m/1 -> Lookup Table (2-D)/1
  Lead-Lag/1 -> Structural Mode Filter/1
  Attitude Gain1/1 -> Transfer Fcn1/1
  rC_rps/1 -> Sum2/2
  Transfer Fcn2/1 -> Sum1/1
  Transfer Fcn1/1 -> Sum1/2
  g2mpss/1 -> Sum2/1

== system AFASClosedloopSim/FMGC (Flight Mgt and Guidance & Control)/AFCC: Albatross.ai Flight Control Computer/FCC: Outerloop & Innerloop Control Laws/HDG Mode/Outerloop Control Law/HDG Flight Director ==
  psiCmd_rad : Inport
  psi_rad : Inport  Port=2
  psiDot_rps : Inport  Port=3
  Attitude Gain1 : Gain  Gain=hdg_select_hdg_rate_track  SaturateOnIntegerOverflow=on  OutDataTypeStr=Inherit: Same as input  ParamDataTypeStr=Inherit: Same as input
      settings: AttributesFormatString=%<Gain>
  Attitude Gain2 : Gain  Gain=hdg_select_hdg_rate_damping  SaturateOnIntegerOverflow=on  OutDataTypeStr=Inherit: Same as input  ParamDataTypeStr=Inherit: Same as input
      settings: AttributesFormatString=%<Gain>
  Attitude Gain3 : Gain  Gain=0.1020  SaturateOnIntegerOverflow=on  OutDataTypeStr=Inherit: Same as input  ParamDataTypeStr=Inherit: Same as input
      settings: AttributesFormatString=1/g
  Constant : Constant  Value=tas_mps
      settings: AttributesFormatString=TAS_mps
  Product : Product  SaturateOnIntegerOverflow=on  OutDataTypeStr=Inherit: Same as first input
  Sum1 : Sum  Inputs=|+-  SaturateOnIntegerOverflow=on
  Sum2 : Sum  Inputs=|+-  SaturateOnIntegerOverflow=on
  phiCmd_rad : Outport
  wires:
  Constant/1 -> Attitude Gain3/1
  Attitude Gain3/1 -> Product/2
  Attitude Gain1/1 -> Product/1
  psi_rad/1 -> Sum2/2
  Product/1 -> Sum1/1
  psiDot_rps/1 -> Attitude Gain2/1
  Attitude Gain2/1 -> Sum1/2
  Sum1/1 -> phiCmd_rad/1
  Sum2/1 -> Attitude Gain1/1
  psiCmd_rad/1 -> Sum2/1

== system AFASClosedloopSim/FMGC (Flight Mgt and Guidance & Control)/AFCC: Albatross.ai Flight Control Computer/FCC: Outerloop & Innerloop Control Laws/HDG Mode/Outerloop Control Law/Roll Command Ay Augmentation ==
  AyAHF_m : Inport
  Attitude Gain3 : Gain  Gain=0.1020  SaturateOnIntegerOverflow=on  OutDataTypeStr=Inherit: Same as input  ParamDataTypeStr=Inherit: Same as input
      settings: AttributesFormatString=1/g
  Gain1 : Gain  Gain=-1  SaturateOnIntegerOverflow=on  OutDataTypeStr=Inherit: Same as input  ParamDataTypeStr=Inherit: Same as input
      settings: AttributesFormatString=Flip Sign
  Transfer Fcn : TransferFcn  Denominator=[lat_accel_aug_lp_tau 1]
      settings: AttributesFormatString=Ay_LP
  augCmd_rad : Outport  InitialOutput=0
  wires:
  AyAHF_m/1 -> Gain1/1
  Attitude Gain3/1 -> Transfer Fcn/1
  Transfer Fcn/1 -> augCmd_rad/1
  Gain1/1 -> Attitude Gain3/1

== system AFASClosedloopSim/FMGC (Flight Mgt and Guidance & Control)/AFCC: Albatross.ai Flight Control Computer/FCC: Outerloop & Innerloop Control Laws/HDG Mode/Outerloop Control Law/Subsystem1 ==
  In : Inport
  ZOH : TransferFcn  Numerator=[-Tau/6 1]  Denominator=[Tau/3 1]
  Out : Outport
  wires:
  In/1 -> ZOH/1
  ZOH/1 -> Out/1

== system AFASClosedloopSim/FMGC (Flight Mgt and Guidance & Control)/AFCC: Albatross.ai Flight Control Computer/FCC: Outerloop & Innerloop Control Laws/HDG Mode/Outerloop Control Law/Subsystem2 ==
  In : Inport
  ZOH : TransferFcn  Numerator=[-Tau/6 1]  Denominator=[Tau/3 1]
  Out : Outport
  wires:
  ZOH/1 -> Out/1
  In/1 -> ZOH/1

== system AFASClosedloopSim/FMGC (Flight Mgt and Guidance & Control)/AFCC: Albatross.ai Flight Control Computer/FCC: Outerloop & Innerloop Control Laws/HDG Mode/Outerloop Control Law/Subsystem3 ==
  In : Inport
  ZOH : TransferFcn  Numerator=[-Tau/6 1]  Denominator=[Tau/3 1]
  Out : Outport
  wires:
  In/1 -> ZOH/1
  ZOH/1 -> Out/1

== system AFASClosedloopSim/FMGC (Flight Mgt and Guidance & Control)/AFCC: Albatross.ai Flight Control Computer/FCC: Outerloop & Innerloop Control Laws/HDG Mode/Outerloop Control Law/Subsystem4 ==
  In : Inport
  ZOH : TransferFcn  Numerator=[-Tau/6 1]  Denominator=[Tau/3 1]
  Out : Outport
  wires:
  ZOH/1 -> Out/1
  In/1 -> ZOH/1

== system AFASClosedloopSim/FMGC (Flight Mgt and Guidance & Control)/AFCC: Albatross.ai Flight Control Computer/FCC: Outerloop & Innerloop Control Laws/HDG Mode/Outerloop Control Law/Subsystem5 ==
  In : Inport
  ZOH : TransferFcn  Numerator=[-Tau/6 1]  Denominator=[Tau/3 1]
  Out : Outport
  wires:
  ZOH/1 -> Out/1
  In/1 -> ZOH/1

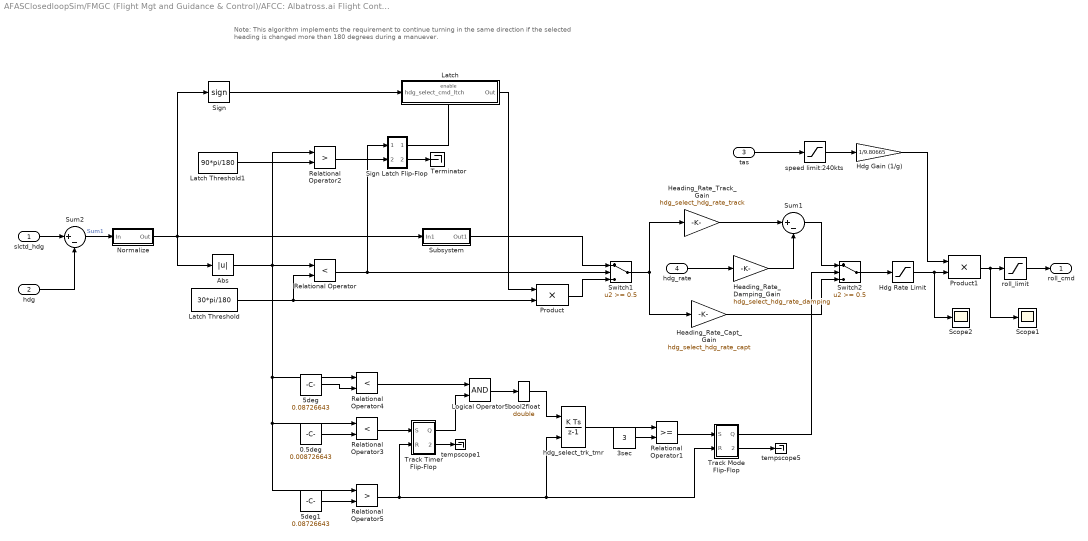
== system AFASClosedloopSim/FMGC (Flight Mgt and Guidance & Control)/AFCC: Albatross.ai Flight Control Computer/FCC: Outerloop & Innerloop Control Laws/HDG Mode/Outerloop Control Law/hdg_select ==
  note: Note: This algorithm implements the requirement to continue turning in the same direction
      |  if the selected heading is changed more than 180 degrees during a manuever.
  slctd_hdg : Inport
  hdg : Inport  Port=2
  tas : Inport  Port=3
  hdg_rate : Inport  Port=4
  0.5deg : Constant  Value=0.008726643
  3sec : Constant  Value=3
  5deg : Constant  Value=0.08726643
  5deg1 : Constant  Value=0.08726643
  Abs : Abs
  Hdg Gain (1/g) : Gain  Gain=1/9.80665  SaturateOnIntegerOverflow=on  OutDataTypeStr=Inherit: Same as input  ParamDataTypeStr=Inherit: Same as input
  Hdg Rate Limit : Saturate  UpperLimit=3*pi/180  LowerLimit=-3*pi/180
  Heading_Rate_Capt_Gain : Gain  Gain=hdg_select_hdg_rate_capt  SaturateOnIntegerOverflow=on  OutDataTypeStr=Inherit: Same as input  ParamDataTypeStr=Inherit: Same as input
  Heading_Rate_Damping_Gain : Gain  Gain=hdg_select_hdg_rate_damping  SaturateOnIntegerOverflow=on  OutDataTypeStr=Inherit: Same as input  ParamDataTypeStr=Inherit: Same as input
  Heading_Rate_Track_Gain : Gain  Gain=hdg_select_hdg_rate_track  SaturateOnIntegerOverflow=on  OutDataTypeStr=Inherit: Same as input  ParamDataTypeStr=Inherit: Same as input
  Latch : Subsystem  TreatAsAtomicUnit=on  RTWFcnName=HDGlatch  RTWFileName=testlatch
      settings: RTWSystemCode=Inline  RTWFcnNameOpts=User specified  RTWFileNameOpts=User specified
  Latch Threshold : Constant  Value=30*pi/180
  Latch Threshold1 : Constant  Value=90*pi/180
  Logical Operator5 : Logic  AllPortsSameDT=off
  Normalize : Subsystem  RTWFcnName=normalize
      settings: RTWFcnNameOpts=User specified
  Product : Product  SaturateOnIntegerOverflow=on  OutDataTypeStr=Inherit: Same as first input
  Product1 : Product  InputSameDT=on  SaturateOnIntegerOverflow=on  OutDataTypeStr=Inherit: Same as first input
  Relational Operator : RelationalOperator  Operator=<  InputSameDT=off
  Relational Operator1 : RelationalOperator  InputSameDT=off
  Relational Operator2 : RelationalOperator  Operator=>  InputSameDT=off
  Relational Operator3 : RelationalOperator  Operator=<  InputSameDT=off
  Relational Operator4 : RelationalOperator  Operator=<  InputSameDT=off
  Relational Operator5 : RelationalOperator  Operator=>  InputSameDT=off
  Scope1 : Scope
  Scope2 : Scope
  Sign : Signum
  Sign Latch Flip-Flop : Subsystem  AncestorBlock=simulink_extras/Flip Flops/S-R Flip-Flop  mask(SRFlipFlop){initial_condition=0}
      mask prompts: initial_condition "Initial condition (state of Q):"
      mask help: S-R Flip-Flop Block
      settings: LibrarySourceBlock=|
      | simulink_extras/Flip Flops/S-R
      | Flip-Flop
      mask Help:
      | The S-R flip-flop also known as a set-reset flip-flop. This implementation
      | is modeled after an S-R flip-flop constructed using NOR gates. The
      | truth table for this block is:
      | <pre>
      |  S  R   Q  !Q
      |  ----------------
      |  1  0   1  0
      |  0  0   1  0  (after S == 1, R == 0)
      |  0  1   0  1
      |  0  0   0  1  (after S == 0, R == 1)
      |  1  1   0  0
      | </pre>
      | 
      | In an S-R flip-flop that is implemented with NOR gates, when a 1 is
      | applied to both the set and reset inputs, both outputs go to 0. Technically,
      | this state is undefined and is usually avoided. Note, if the flip-flop is
      | implemented with NAND gates, when a 0 is applied to both inputs, both outputs
      | go to 0 and when a 1 is applied to both inputs, the output depends on
      | the previous state of the flip-flop (previous value of Q).
  Subsystem : Subsystem
  Sum1 : Sum  Inputs=|+-  InputSameDT=on  SaturateOnIntegerOverflow=on  OutDataTypeStr=Inherit: Same as first input
  Sum2 : Sum  Inputs=|+-  InputSameDT=on  SaturateOnIntegerOverflow=on  OutDataTypeStr=Inherit: Same as first input
  Switch1 : Switch  Threshold=0.5  InputSameDT=off
  Switch2 : Switch  Threshold=0.5  InputSameDT=off
  Terminator : Terminator
  Track Mode Flip-Flop : Subsystem  AncestorBlock=simulink_extras/Flip Flops/S-R Flip-Flop  mask(SRFlipFlop){initial_condition=0}
      mask prompts: initial_condition "Initial condition (state of Q):"
      mask help: S-R Flip-Flop Block
      settings: LibrarySourceBlock=|
      | simulink_extras/Flip Flops/S-R
      | Flip-Flop
      mask Help:
      | The S-R flip-flop also known as a set-reset flip-flop. This implementation
      | is modeled after an S-R flip-flop constructed using NOR gates. The
      | truth table for this block is:
      | <pre>
      |  S  R   Q  !Q
      |  ----------------
      |  1  0   1  0
      |  0  0   1  0  (after S == 1, R == 0)
      |  0  1   0  1
      |  0  0   0  1  (after S == 0, R == 1)
      |  1  1   0  0
      | </pre>
      | 
      | In an S-R flip-flop that is implemented with NOR gates, when a 1 is
      | applied to both the set and reset inputs, both outputs go to 0. Technically,
      | this state is undefined and is usually avoided. Note, if the flip-flop is
      | implemented with NAND gates, when a 0 is applied to both inputs, both outputs
      | go to 0 and when a 1 is applied to both inputs, the output depends on
      | the previous state of the flip-flop (previous value of Q).
  Track Timer Flip-Flop : Subsystem  AncestorBlock=simulink_extras/Flip Flops/S-R Flip-Flop  mask(SRFlipFlop){initial_condition=0}
      mask prompts: initial_condition "Initial condition (state of Q):"
      mask help: S-R Flip-Flop Block
      settings: LibrarySourceBlock=|
      | simulink_extras/Flip Flops/S-R
      | Flip-Flop
      mask Help:
      | The S-R flip-flop also known as a set-reset flip-flop. This implementation
      | is modeled after an S-R flip-flop constructed using NOR gates. The
      | truth table for this block is:
      | <pre>
      |  S  R   Q  !Q
      |  ----------------
      |  1  0   1  0
      |  0  0   1  0  (after S == 1, R == 0)
      |  0  1   0  1
      |  0  0   0  1  (after S == 0, R == 1)
      |  1  1   0  0
      | </pre>
      | 
      | In an S-R flip-flop that is implemented with NOR gates, when a 1 is
      | applied to both the set and reset inputs, both outputs go to 0. Technically,
      | this state is undefined and is usually avoided. Note, if the flip-flop is
      | implemented with NAND gates, when a 0 is applied to both inputs, both outputs
      | go to 0 and when a 1 is applied to both inputs, the output depends on
      | the previous state of the flip-flop (previous value of Q).
  bool2float : DataTypeConversion  OutDataTypeStr=double
  hdg_select_trk_tmr : DiscreteIntegrator  ExternalReset=rising  SampleTime=0.1  LimitOutput=on  UpperSaturationLimit=4  LowerSaturationLimit=0  ICPrevOutput=DiscIntNeverNeededParam  ICPrevScaledInput=DiscIntNeverNeededParam
  roll_limit : Saturate  UpperLimit=roll_limit  LowerLimit=-roll_limit
  speed limit:240kts : Saturate  UpperLimit=123.4667  LowerLimit=0.0
  tempscope1 : Terminator
  tempscope5 : Terminator
  roll_cmd : Outport  InitialOutput=0
  wires:
  hdg/1 -> Sum2/2
  Hdg Rate Limit/1 -> Product1/2, Scope2/1
  Switch2/1 -> Hdg Rate Limit/1
  tas/1 -> speed limit:240kts/1
  Hdg Gain (1/g)/1 -> Product1/1
  Sum2/1 -> Normalize/1(In)  "Sum1"
  Normalize/1(Out) -> Subsystem/1(In1), Abs/1, Sign/1
  Abs/1 -> Relational Operator/1, Relational Operator4/1, Relational Operator3/1, Relational Operator5/1, Relational Operator2/1
  Latch Threshold/1 -> Relational Operator/2, Product/2
  Relational Operator/1 -> Switch1/2, Sign Latch Flip-Flop/1(S)
  Product1/1 -> roll_limit/1, Scope1/1
  Switch1/1 -> Heading_Rate_Capt_Gain/1, Heading_Rate_Track_Gain/1
  Sign/1 -> Latch/1(hdg_select_cmd_ltch)
  Product/1 -> Switch1/3
  slctd_hdg/1 -> Sum2/1
  Latch/1(Out) -> Product/1
  Subsystem/1(Out1) -> Switch1/1
  speed limit:240kts/1 -> Hdg Gain (1/g)/1
  Latch Threshold1/1 -> Relational Operator2/2
  Relational Operator2/1 -> Sign Latch Flip-Flop/2(R)
  Sign Latch Flip-Flop/1(Q) -> Latch/Enable
  Sign Latch Flip-Flop/2(!Q) -> Terminator/1
  3sec/1 -> Relational Operator1/2
  hdg_select_trk_tmr/1 -> Relational Operator1/1
  Relational Operator1/1 -> Track Mode Flip-Flop/1(S)
  0.5deg/1 -> Relational Operator3/2
  Relational Operator3/1 -> Track Timer Flip-Flop/1(S)
  5deg/1 -> Relational Operator4/2
  Relational Operator4/1 -> Logical Operator5/1
  Logical Operator5/1 -> bool2float/1
  Track Mode Flip-Flop/2(!Q) -> tempscope5/1
  Track Mode Flip-Flop/1(Q) -> Switch2/2
  Heading_Rate_Capt_Gain/1 -> Switch2/3
  5deg1/1 -> Relational Operator5/2
  Relational Operator5/1 -> Track Mode Flip-Flop/2(R), hdg_select_trk_tmr/2, Track Timer Flip-Flop/2(R)
  Track Timer Flip-Flop/1(Q) -> Logical Operator5/2
  Track Timer Flip-Flop/2(!Q) -> tempscope1/1
  bool2float/1 -> hdg_select_trk_tmr/1
  Heading_Rate_Track_Gain/1 -> Sum1/1
  Sum1/1 -> Switch2/1
  hdg_rate/1 -> Heading_Rate_Damping_Gain/1
  Heading_Rate_Damping_Gain/1 -> Sum1/2
  roll_limit/1 -> roll_cmd/1

== system AFASClosedloopSim/FMGC (Flight Mgt and Guidance & Control)/AFCC: Albatross.ai Flight Control Computer/FCC: Outerloop & Innerloop Control Laws/HDG Mode/Innerloop Control Law/Roll AP/Autopilot IAS-scheduled Gain ==
  ias : Inport
  Look-Up Table : Lookup  InputValues="[ias_1  ias_2]"  Table="[abs_gain_1  abs_gain_2]"  LookUpMeth=Interpolation-Use End Values
  Product : Product  InputSameDT=on  SaturateOnIntegerOverflow=on  OutDataTypeStr=Inherit: Same as first input
  dB->linear : Fcn  Expr=2^(u(1)/8)
  gain sign : Constant
  scheduled_gain : Outport
  wires:
  Look-Up Table/1 -> dB->linear/1
  dB->linear/1 -> Product/1
  ias/1 -> Look-Up Table/1
  Product/1 -> scheduled_gain/1
  gain sign/1 -> Product/2

== system AFASClosedloopSim/FMGC (Flight Mgt and Guidance & Control)/AFCC: Albatross.ai Flight Control Computer/FCC: Outerloop & Innerloop Control Laws/HDG Mode/Innerloop Control Law/YD Control Law/Autopilot IAS-scheduled Gain ==
  note: gain sign
  ias : Inport
  Constant : Constant
  Look-Up Table : Lookup  InputValues="[ias_1  ias_2]"  Table="[abs_gain_1  abs_gain_2]"  LookUpMeth=Interpolation-Use End Values
  Product : Product  InputSameDT=on  SaturateOnIntegerOverflow=on  OutDataTypeStr=Inherit: Same as first input
  dB->linear : Fcn  Expr=2^(u(1)/8)
  scheduled_gain : Outport
  wires:
  Look-Up Table/1 -> dB->linear/1
  dB->linear/1 -> Product/1
  ias/1 -> Look-Up Table/1
  Product/1 -> scheduled_gain/1
  Constant/1 -> Product/2

== system AFASClosedloopSim/FMGC (Flight Mgt and Guidance & Control)/AFCC: Albatross.ai Flight Control Computer/FCC: Outerloop & Innerloop Control Laws/HDG Mode/Outerloop Control Law/hdg_select/Latch ==
  hdg_select_cmd_ltch : Inport
  Enable : EnablePort
  Out : Outport  InitialOutput=0
  wires:
  hdg_select_cmd_ltch/1 -> Out/1

== system AFASClosedloopSim/FMGC (Flight Mgt and Guidance & Control)/AFCC: Albatross.ai Flight Control Computer/FCC: Outerloop & Innerloop Control Laws/HDG Mode/Outerloop Control Law/hdg_select/Normalize ==
  note: Normalize Angle
  In : Inport
  Constant : Constant  Value=pi
  Constant1 : Constant  Value=2*pi
  Constant2 : Constant  Value=-pi
  Constant3 : Constant  Value=0
  Relational Operator : RelationalOperator  InputSameDT=off
  Relational Operator1 : RelationalOperator  Operator=<  InputSameDT=off
  Sum : Sum  Inputs=++-  SaturateOnIntegerOverflow=on
  Switch : Switch  Threshold=0.5  InputSameDT=off
  Switch1 : Switch  Threshold=0.5  InputSameDT=off
  Out : Outport
  wires:
  In/1 -> Sum/2, Relational Operator/1, Relational Operator1/1
  Constant/1 -> Relational Operator/2
  Sum/1 -> Out/1  "NormalizedAngle"
  Constant2/1 -> Relational Operator1/2
  Constant1/1 -> Switch/1, Switch1/1
  Relational Operator/1 -> Switch/2
  Constant3/1 -> Switch1/3, Switch/3
  Switch1/1 -> Sum/1
  Switch/1 -> Sum/3
  Relational Operator1/1 -> Switch1/2

== system AFASClosedloopSim/FMGC (Flight Mgt and Guidance & Control)/AFCC: Albatross.ai Flight Control Computer/FCC: Outerloop & Innerloop Control Laws/HDG Mode/Outerloop Control Law/hdg_select/Sign Latch Flip-Flop ==
  S : Inport
  R : Inport  Port=2
  Demux : Demux  Outputs=2
      settings: DisplayOption=none
  Logic : CombinatorialLogic  TruthTable=[0 1;1 0;0 1;0 1;1 0;1 0;0 0;0 0]
  Mux : Mux  Inputs=3
  hdg_select_latch : Memory  InitialCondition=initial_condition  InheritSampleTime=on
  Q : Outport  InitialOutput=0
  !Q : Outport  Port=2  InitialOutput=1
  wires:
  hdg_select_latch/1 -> Mux/3
  Mux/1 -> Logic/1
  Logic/1 -> Demux/1
  Demux/2 -> !Q/1
  Demux/1 -> Q/1, hdg_select_latch/1
  S/1 -> Mux/1
  R/1 -> Mux/2

== system AFASClosedloopSim/FMGC (Flight Mgt and Guidance & Control)/AFCC: Albatross.ai Flight Control Computer/FCC: Outerloop & Innerloop Control Laws/HDG Mode/Outerloop Control Law/hdg_select/Subsystem ==
  In1 : Inport
  Sum1 : Sum  Inputs=|+-  InputSameDT=on  SaturateOnIntegerOverflow=on  OutDataTypeStr=Inherit: Same as first input
  Sum2 : Sum  Inputs=|++  InputSameDT=on  SaturateOnIntegerOverflow=on  OutDataTypeStr=Inherit: Same as first input
  hdg_select_gain : Gain  Gain=0.5  SaturateOnIntegerOverflow=on  OutDataTypeStr=Inherit: Same as input  ParamDataTypeStr=Inherit: Same as input
  hdg_select_hdg_swtch : Saturate  UpperLimit=5*pi/180  LowerLimit=-5*pi/180
  Out1 : Outport
  wires:
  In1/1 -> hdg_select_hdg_swtch/1, Sum1/1
  hdg_select_hdg_swtch/1 -> Sum1/2, Sum2/2
  Sum1/1 -> hdg_select_gain/1
  hdg_select_gain/1 -> Sum2/1
  Sum2/1 -> Out1/1

== system AFASClosedloopSim/FMGC (Flight Mgt and Guidance & Control)/AFCC: Albatross.ai Flight Control Computer/FCC: Outerloop & Innerloop Control Laws/HDG Mode/Outerloop Control Law/hdg_select/Track Mode Flip-Flop ==
  S : Inport
  R : Inport  Port=2
  Demux : Demux  Outputs=2
      settings: DisplayOption=none
  Logic : CombinatorialLogic  TruthTable=[0 1;1 0;0 1;0 1;1 0;1 0;0 0;0 0]
  Mux : Mux  Inputs=3
  hdg_select_trk : Memory  InitialCondition=initial_condition  InheritSampleTime=on
  Q : Outport  InitialOutput=0
  !Q : Outport  Port=2  InitialOutput=1
  wires:
  hdg_select_trk/1 -> Mux/3
  Mux/1 -> Logic/1
  Logic/1 -> Demux/1
  Demux/2 -> !Q/1
  Demux/1 -> Q/1, hdg_select_trk/1
  S/1 -> Mux/1
  R/1 -> Mux/2

== system AFASClosedloopSim/FMGC (Flight Mgt and Guidance & Control)/AFCC: Albatross.ai Flight Control Computer/FCC: Outerloop & Innerloop Control Laws/HDG Mode/Outerloop Control Law/hdg_select/Track Timer Flip-Flop ==
  S : Inport
  R : Inport  Port=2
  Demux : Demux  Outputs=2
      settings: DisplayOption=none
  Logic : CombinatorialLogic  TruthTable=[0 1;1 0;0 1;0 1;1 0;1 0;0 0;0 0]
  Mux : Mux  Inputs=3
  hdg_select_timer : Memory  InitialCondition=initial_condition  InheritSampleTime=on
  Q : Outport  InitialOutput=0
  !Q : Outport  Port=2  InitialOutput=1
  wires:
  R/1 -> Mux/2
  S/1 -> Mux/1
  Demux/1 -> hdg_select_timer/1, Q/1
  Demux/2 -> !Q/1
  Logic/1 -> Demux/1
  Mux/1 -> Logic/1
  hdg_select_timer/1 -> Mux/3

== matlab function AFASClosedloopSim/AFAS has four sub-moduels: 1) Detect and Avoid (DAA); 2) Aircraft Separation Assurance System (ASAS); 3) Collaborative Decision Assistance System (CDAS); 4) Decentralized Decision Assistance System (DDAS) /DDAS: Decentralized Decision Assistance System/If Action Subsystem1/Optimize Function ==
  data: separationTime input; data input; AwarenessETA input; t output; s output; ownshipETA input; over output
function [t,s,over]= Optimize(separationTime, data, AwarenessETA, ownshipETA)
%#codegen
t=[0,0,0,0,0,0,0];
s=zeros(7,7);
coder.extrinsic('optimizeFunction')
if(data~=1)
[t,s]=  optimizeFunction(separationTime, AwarenessETA, ownshipETA);
over=1;
else
    over=1;
end

== stateflow chart AFASClosedloopSim/AFAS has four sub-moduels: 1) Detect and Avoid (DAA); 2) Aircraft Separation Assurance System (ASAS); 3) Collaborative Decision Assistance System (CDAS); 4) Decentralized Decision Assistance System (DDAS) /DDAS: Decentralized Decision Assistance System/Chart ==
  state Active
    entry:
    sessionState=1;
    state Engaged
      state Locked
        entry:
        sessionState=3;
      state Scheduling
        entry:
        sessionState=4;
      state Unlock
        entry:
        sessionState=5;
      (default) -> Locked
      Locked -> Scheduling [order 2] : after(10,sec)
      Scheduling -> Unlock [order 2] : [confirmData==1]
    state Preparation
      entry:
      sessionState=2;
    (default) -> Preparation
    Preparation -> Engaged : after(10,sec)
  state Initialization
    entry:
    sessionState=0;
  state Pause
    entry:
    sessionState=7;
  state TimeOut
    entry:
    sessionState=6;
  Unlock -> Initialization : after(10,sec)
  (default) -> Initialization
  Initialization -> Active [order 2] : [InRange==1 && confirmData==0]
  Active -> Initialization : [sessionState==5]
  Initialization -> Pause [order 1] : [Pause==1]
  Pause -> Initialization : [Pause==0]
  TimeOut -> Initialization : after(10,sec)
  Locked -> TimeOut [order 1] : after(20,sec)
  Scheduling -> TimeOut [order 1] : after(20,sec)
  data: confirmData input; InRange input; sessionState output; Pause input

== stateflow chart AFASClosedloopSim/SA Initialization /Chart1 ==
  state Sensing
    entry:
    Sensed=0;
  state In
    entry:
    Sensed=1;
  (default) -> Sensing
  Sensing -> In : [InScope==1]
  data: Sensed output =0; InScope input; data1 input; green local =1; red local =0; yellow local =0; fault local =0; data input
